simulink model "P2d_salidas"  (R2014a)
settings: Solver=ode45  StartTime=0.0  StopTime=1200  RelTol=1e-3
undefined symbols (not defined in the file): beta, c1, c2, h_high_cm, h_low_cm, h_mid_cm, idss, k1_high, k1_low, k1_mid, k2_high, k2_low, k2_mid, modelo_lineal_rango_alto, modelo_lineal_rango_bajo, modelo_lineal_rango_medio, u_high, u_low
libraries: slident x3
settings Model: Creator=matias  LastModifiedBy=pdoren
settings DataIOCC: SignalLoggingSaveFormat=ModelDataLogs
settings OptimizationCC: ExpressionDepthLimit=2147483647
settings DebuggingCC: UnderspecifiedInitializationDetection=Classic  FcnCallInpInsideContextMsg=EnableAllAsWarning  StateNameClashWarn=warning

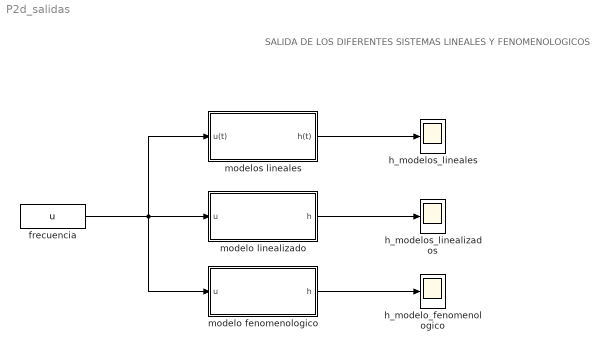
== system P2d_salidas ==
  note: SALIDA DE LOS DIFERENTES SISTEMAS LINEALES Y FENOMENOLOGICOS
  frecuencia : FromWorkspace  VariableName=u  SampleTime=0
  h_modelo_fenomenologico : Scope
      settings: TimeRange=1200  YMin=22.6  YMax=25  SaveName=h_modelo_fenomenologico
  h_modelos_lineales : Scope
      settings: TimeRange=1200  YMin=22.6  YMax=25  SaveName=h_modelos_lineales
  h_modelos_linealizados : Scope
      settings: TimeRange=1200  YMin=22.6  YMax=25  SaveName=h_modelos_linealizados
  modelo fenomenologico : Subsystem  Tag=Modelo Fenomenologico
  modelo linealizado : Subsystem  Tag=Modelo Fenomenologico
  modelos lineales : Subsystem  Tag=Modelo Fenomenologico
  wires:
  modelos lineales/1(h(t)) -> h_modelos_lineales/1
  modelo fenomenologico/1(h) -> h_modelo_fenomenologico/1
  modelo linealizado/1(h) -> h_modelos_linealizados/1
  frecuencia/1 -> modelo linealizado/1(u), modelo fenomenologico/1(u), modelos lineales/1(u(t))

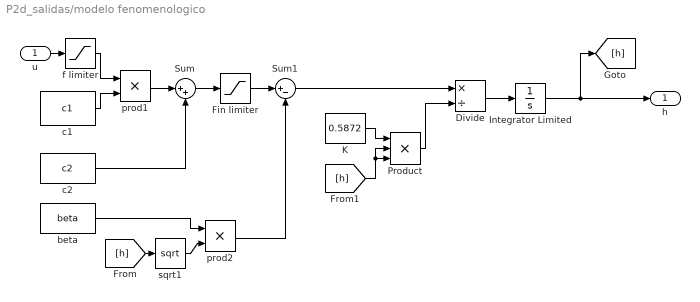
== system P2d_salidas/modelo fenomenologico ==
  u : Inport
  Divide : Product  Inputs=*/
  Fin limiter : Saturate  UpperLimit=inf  LowerLimit=0
  Integrator Limited : Integrator  InitialCondition=0.1  LimitOutput=on  UpperSaturationLimit=80  LowerSaturationLimit=0.1
  K : Constant  Value=0.5872
  Product : Product  Inputs=3  RndMeth=Zero
  Sum : Sum  Inputs=|++
  Sum1 : Sum  Inputs=|+-
  beta : Constant  Value=beta
  c1 : Constant  Value=c1
  c2 : Constant  Value=c2
  f limiter : Saturate  UpperLimit=100  LowerLimit=0
  prod1 : Product  RndMeth=Zero
  prod2 : Product  RndMeth=Zero
  sqrt1 : Sqrt  SaturateOnIntegerOverflow=on
  h : Outport
  wires:
  f limiter/1 -> prod1/1
  c1/1 -> prod1/2
  prod1/1 -> Sum/1
  c2/1 -> Sum/2
  beta/1 -> prod2/1
  prod2/1 -> Sum1/2
  sqrt1/1 -> prod2/2
  Sum1/1 -> Divide/1
  [h] -> sqrt1/1
  Product/1 -> Divide/2
  K/1 -> Product/1
  [h] -> Product/2, Product/3
  Divide/1 -> Integrator Limited/1
  Integrator Limited/1 -> h/1, [h]
  Sum/1 -> Fin limiter/1
  Fin limiter/1 -> Sum1/1
  u/1 -> f limiter/1

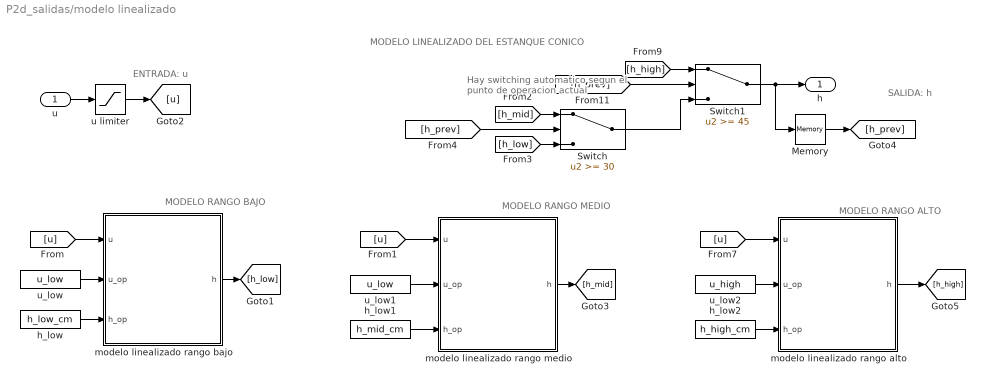
== system P2d_salidas/modelo linealizado ==
  note: MODELO RANGO BAJO
  note: MODELO RANGO MEDIO
  note: MODELO RANGO ALTO
  note: ENTRADA: u
  note: MODELO LINEALIZADO DEL ESTANQUE CONICO
  note: Hay switching automatico segun
      | el punto de operacion actual
  note: SALIDA: h
  u : Inport
  Memory : Memory
  Switch : Switch  Threshold=30
  Switch1 : Switch  Threshold=45
  h_low : Constant  Value=h_low_cm
  h_low1 : Constant  Value=h_mid_cm
  h_low2 : Constant  Value=h_high_cm
  modelo linealizado rango alto : Subsystem
  modelo linealizado rango bajo : Subsystem
  modelo linealizado rango medio : Subsystem
  u limiter : Saturate  UpperLimit=100  LowerLimit=0
  u_low : Constant  Value=u_low
  u_low1 : Constant  Value=u_low
  u_low2 : Constant  Value=u_high
  h : Outport
  wires:
  u/1 -> u limiter/1
  u_low/1 -> modelo linealizado rango bajo/2(u_op)
  h_low/1 -> modelo linealizado rango bajo/3(h_op)
  modelo linealizado rango bajo/1(h) -> [h_low]
  u limiter/1 -> [u]
  [u] -> modelo linealizado rango bajo/1(u)
  modelo linealizado rango medio/1(h) -> [h_mid]
  [h_mid] -> Switch/1
  [h_low] -> Switch/3
  Memory/1 -> [h_prev]
  [h_prev] -> Switch/2
  u_low2/1 -> modelo linealizado rango alto/2(u_op)
  h_low2/1 -> modelo linealizado rango alto/3(h_op)
  modelo linealizado rango alto/1(h) -> [h_high]
  [u] -> modelo linealizado rango alto/1(u)
  [h_high] -> Switch1/1
  Switch/1 -> Switch1/3
  [h_prev] -> Switch1/2
  Switch1/1 -> h/1, Memory/1
  [u] -> modelo linealizado rango medio/1(u)
  u_low1/1 -> modelo linealizado rango medio/2(u_op)
  h_low1/1 -> modelo linealizado rango medio/3(h_op)

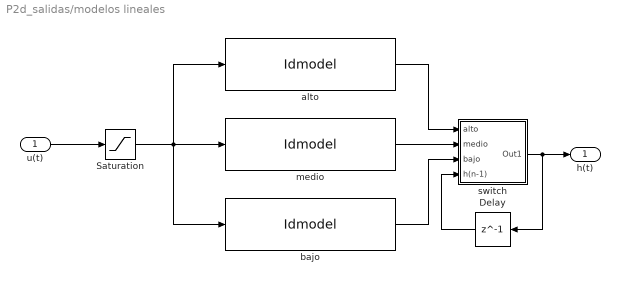
== system P2d_salidas/modelos lineales ==
  u(t) : Inport
  Delay : Delay  DelayLength=1
  Saturation : Saturate  UpperLimit=100  LowerLimit=0
  alto : slident/Models/Idmodel  sys=idss(modelo_lineal_rango_alto)  IC=X0_alto  noi=on  seed=[]
  bajo : slident/Models/Idmodel  sys=idss(modelo_lineal_rango_bajo)  IC=X0_bajo  noi=on  seed=[]
  medio : slident/Models/Idmodel  sys=idss(modelo_lineal_rango_medio)  IC=X0_medio  noi=on  seed=[]
  switch : Subsystem
  h(t) : Outport
  wires:
  medio/1 -> switch/2(medio)
  switch/1(Out1) -> h(t)/1, Delay/1
  bajo/1 -> switch/3(bajo)
  alto/1 -> switch/1(alto)
  u(t)/1 -> Saturation/1
  Saturation/1 -> bajo/1, alto/1, medio/1
  Delay/1 -> switch/4(h(n-1))

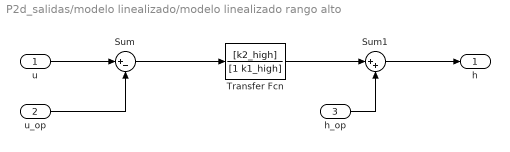
== system P2d_salidas/modelo linealizado/modelo linealizado rango alto ==
  u : Inport
  u_op : Inport  Port=2
  h_op : Inport  Port=3
  Sum : Sum  Inputs=|+-
  Sum1 : Sum  Inputs=|++
  Transfer Fcn : TransferFcn  Numerator=[k2_high]  Denominator=[1 k1_high]
  h : Outport
  wires:
  u_op/1 -> Sum/2
  Sum1/1 -> h/1
  h_op/1 -> Sum1/2
  u/1 -> Sum/1
  Sum/1 -> Transfer Fcn/1
  Transfer Fcn/1 -> Sum1/1

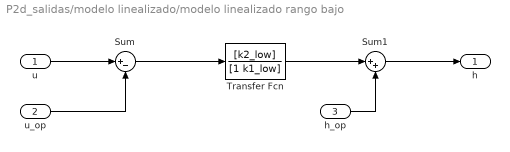
== system P2d_salidas/modelo linealizado/modelo linealizado rango bajo ==
  u : Inport
  u_op : Inport  Port=2
  h_op : Inport  Port=3
  Sum : Sum  Inputs=|+-
  Sum1 : Sum  Inputs=|++
  Transfer Fcn : TransferFcn  Numerator=[k2_low]  Denominator=[1 k1_low]
  h : Outport
  wires:
  u_op/1 -> Sum/2
  Sum1/1 -> h/1
  h_op/1 -> Sum1/2
  u/1 -> Sum/1
  Sum/1 -> Transfer Fcn/1
  Transfer Fcn/1 -> Sum1/1

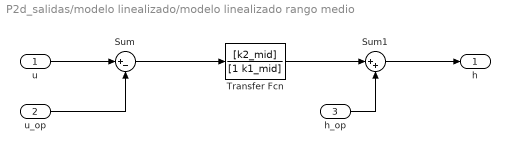
== system P2d_salidas/modelo linealizado/modelo linealizado rango medio ==
  u : Inport
  u_op : Inport  Port=2
  h_op : Inport  Port=3
  Sum : Sum  Inputs=|+-
  Sum1 : Sum  Inputs=|++
  Transfer Fcn : TransferFcn  Numerator=[k2_mid]  Denominator=[1 k1_mid]
  h : Outport
  wires:
  u_op/1 -> Sum/2
  Sum1/1 -> h/1
  h_op/1 -> Sum1/2
  u/1 -> Sum/1
  Sum/1 -> Transfer Fcn/1
  Transfer Fcn/1 -> Sum1/1

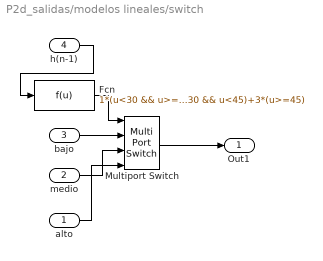
== system P2d_salidas/modelos lineales/switch ==
  alto : Inport
  medio : Inport  Port=2
  bajo : Inport  Port=3
  h(n-1) : Inport  Port=4
  Fcn : Fcn  Expr=1*(u<30 && u>=0)+2*(u>=30 && u<45)+3*(u>=45)
  Multiport Switch : MultiPortSwitch
  Out1 : Outport
  wires:
  Multiport Switch/1 -> Out1/1
  bajo/1 -> Multiport Switch/2
  medio/1 -> Multiport Switch/3
  alto/1 -> Multiport Switch/4
  Fcn/1 -> Multiport Switch/1
  h(n-1)/1 -> Fcn/1
